simulink model "i_128w_2k_10_r306f"  (Simulink 7.0)
settings: Solver=ode45  StartTime=0.0  StopTime=100000  RelTol=1e-3
undefined symbols (not defined in the file or in its folder): iBOB, pfb_coeff_gen_calc
libraries: xbsIndex_r4 x946, casper_library x68, xps_library x29, xbsReplacements_r4 x12, simulink x1
(part 1 of 10)
settings Model: Creator=dsp  LastModifiedBy=dsp

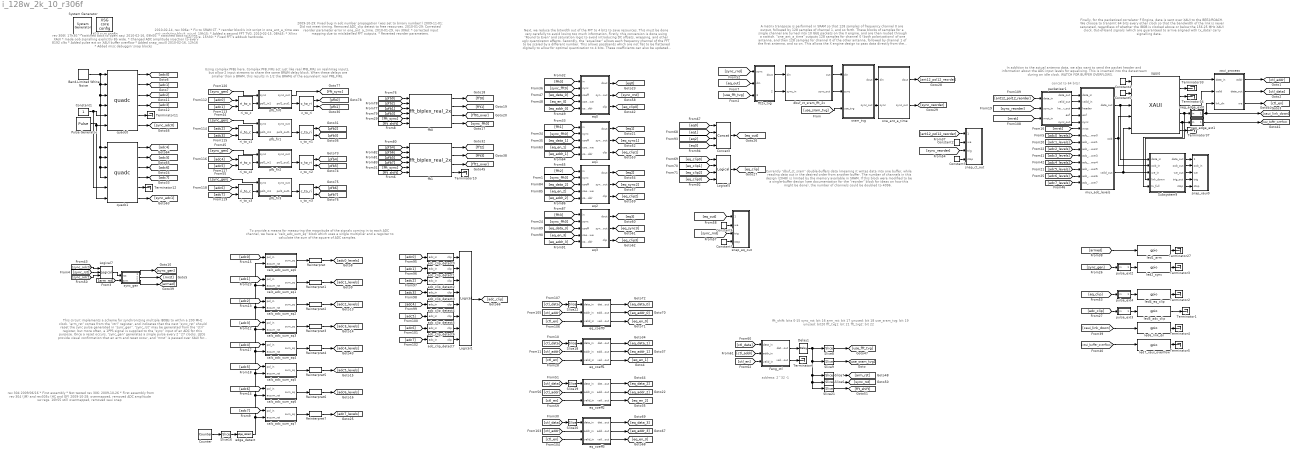
== system i_128w_2k_10_r306f ==
  note: 2010-02-14, rev 306e:
      |   * Fix to SRAM CT.
      |   * reorder block's init script in one_ant_a_time was not updating block. wierd.
      | 19h15:
      |   * Added a second FFT TVG.
      | 2010-02-15, 08h45:
      |   * Xilinx XAUI core.
      | 15h30:
      |   * Fixed FFT's addsub hardcode.
  note: This circuit implements a scheme for synchronizing
      | multiple IBOBs to within a 200 MHz clock.  "arm_rst"
      | comes from the "ctrl" register, and indicates that the
      | next "sync_rst" should reset the sync pulse generated
      | in "sync_gen".  "sync_rst" may be generated from
      | the "ctrl" register, but more often, a 1PPS signal is
      | supplied to the "sync" input of an ADC for this
      | purpose.  Once a reset occurs, "sync_gen" generates
      | a single pulse every 2^27 clocks.  LEDs provide visual
      | confirmation that an arm and reset occur, and "mrst"
      | is passed over XAUI for the purpose of informing
      | downstream logic in a packetized correlator that
      | a "master reset" has occurred.
  note: Using complex PFBs here.  Complex PFB_FIRs act just like real
      | PFB_FIRs on real/imag inputs, but  allow 2 input streams to
      | share the same BRAM delay block.  When these delays are smaller
      | than a BRAM, this results in 1/2 the BRAMs of the equivalent real
      | PFB_FIRs.
  note: To provide a means for measuring the magnitude of the signals
      | coming in to each ADC channel, we have a "calc_adc_sum_sq"
      | block which uses a single multiplier and a regsiter to calculate
      | the sum of the square of ADC samples.
  note: fft_shift: bits 0-15
      | sync_rst: bit 16
      | arm_rst: bit 17
      | unused: bit 18
      | use_sram_tvg: bit 19
      | unused: bit20
      | fft_tvg1: bit 21
      | fft_tvg2: bit 22
  note: address: 2^32 -1
  note: Finally, for the packetized correlator F Engine, data is sent over
      | XAUI to the BEE2/ROACH.  We choose to transmit 64 bits every other clock
      | so that the bandwidth of the link is never saturated, regardless of whether
      | the IBOB is clocked above or below the 156.25 MHz XAUI clock.
      | Out-of-band signals (which are guaranteed to arrive aligned with
      | tx_data) carry signalling data.
  note: In addition to the actual antenna data,
      | we also want to send the packet header
      | and information about the ADC input levels for equalising.
      | This is inserted into the datastream during an idle clock.
      | WATCH FOR BUFFER OVERFLOWS.
  note: concat to 64 bits!
  note: A matrix transpose is performed in SRAM so that 128 samples of frequency
      | channel 0 are output, followed by 128 samples of channel 1, and so forth.
      | These blocks of samples for a single channel are turned into 10 GbE packets
      | on the X engine, and are then routed through a swittch.  "one_ant_a_time"
      | outputs 128 samples for channel 0 (both polarizations) of one antenna,
      | and then 128 samples for channel 0 of the other antenna, followed by
      | channel 1 of the first antenna, and so on.  This allows the X engine design to
      | pass data directly from the XAUI into a packet containing 128 time samples
      | for 1 frequency from 1 antenna.
  note: Currently "dbuf_ct_sram" double-buffers data (meaning it writes data
      | into one buffer, while reading data out in the desired order from another
      | buffer.  The number of channels in this design (2048) is limited by the
      | memory available in SRAM.  If this block were modified to be a
      | single-buffer design (see documentation for the "reorder" block for
      | ideas on how this might be done), the number of channels could
      | be doubled to 4096.
  note: Next, we reduce the bitwidth out of the FFT to 4 bits to save resources.
      | This must be done very carefully to avoid losing too much information.
      | Firstly, this conversion is done using "Round to Even" and saturation
      | logic to avoid introducing DC offsets, wrapping, and other ugly quantizaton
      | effects.  Secondly, the "equalizer" allows each frequency channel of the
      | FFT to be scaled by a different number.  This allows passbands which are
      | not flat to be flattened digitally to allow for optimal quantization to 4 bits.
      | These coefficients can also be updated dynamically for gain control.
      | Coefficients can be dynamically written into the "equalizer" by
      | specifying the channel ("coeff_addr") and the value of the
      | coefficient ("coeff"), and then using "coeff_en" to write the
      | new coefficient into the equalization table.
  note: rev 304 2009/06/16
      | * First assembly
      | * Not tested
      |
      | rev 306: 2009-10-26
      | * First assembly from rev 304 (JM) and rev305c (HC and GF)
      |
      | 2009-10-28: overmapped, removed ADC amplitude sw regs.
      | 10h55 still overmapped, removed xaui snap
  note: 2009-10-29: Fixed bug in adc number propagation (was set to binary number!)
      | 2009-11-01: Did not meet timing. Removed ADC_clip detect to free resources.
      | 2010-01-29: Corrected reorder parameter error in one_ant_a_time.
      |
      | 2010-01-29, rev 306d:
      |   * corrected input mapping due to mislabelled FFT outputs.
      |   * Reverted reorder parameters.
  note: rev 306f, 17h30:
      |   * switched back to open xaui
      | 2010-02-16, 09h00:
      |   * switched back to Xilinx XAUI
      |   * made oob signalling explicitly 8b wide.
      |   * Changed ADC amplitude injection to every 8192 clks
      |   * Added pulse ext on XAUI buffer overflow
      |   * Added snap_xaui0
      | 2010-02-16, 12h16
      |   * Added misc debuggin' snap blocks
  " System Generator" : xbsIndex_r4/ System Generator  Tag=genX  SystemSampleTime=-1  xilinxfamily=virtex2p  part=xc2vp50  speed=-7  package=ff1152  synthesis_tool=XST  clock_wrapper=Clock Enables  directory=./i_128w_2k_10_r306f/sysgen  testbench=off  simulink_period=1  sysclk_period=5  dcm_input_clock_period=100  incr_netlist=off  trim_vbits=Everywhere in SubSystem  dbl_ovrd=According to Block Masks  core_generation=According to Block Masks  run_coregen=off  deprecated_control=off  eval_field=0  block_type=sysgen
      settings: block_version=10.1.3
  Band-Limited White Noise : simulink/Sources/Band-Limited White Noise  SystemSampleTime=-1  Cov=[0.1]  Ts=0.1  seed=[23341]
  Concat3 : xbsIndex_r4/Concat  num_inputs=4  dbl_ovrd=off  block_type=concat
      settings: block_version=10.1.3
  Constant1 : Constant  OutDataType=sfix(16)  OutScaling=2^0
  Constant2 : xbsIndex_r4/Constant  arith_type=Boolean  const=1  n_bits=1  bin_pt=0  explicit_period=on  period=1  equ=P=C  opselect=C  inp2=PCIN>>17  opr=+  inp1=P  carry=CIN  dbl_ovrd=off  block_type=constant
  Constant3 : xbsIndex_r4/Constant  arith_type=Boolean  const=0  n_bits=1  bin_pt=0  explicit_period=on  period=1  equ=P=C  opselect=C  inp2=PCIN>>17  opr=+  inp1=P  carry=CIN  dbl_ovrd=off  block_type=constant
  Constant4 : xbsIndex_r4/Constant  arith_type=Unsigned  const=1  n_bits=1  bin_pt=0  explicit_period=on  period=1  equ=P=C  opselect=C  inp2=PCIN>>17  opr=+  inp1=P  carry=CIN  dbl_ovrd=off  block_type=constant
  Constant5 : xbsIndex_r4/Constant  arith_type=Unsigned  const=0  n_bits=1  bin_pt=0  explicit_period=on  period=1  equ=P=C  opselect=C  inp2=PCIN>>17  opr=+  inp1=P  carry=CIN  dbl_ovrd=off  block_type=constant
  Constant6 : xbsIndex_r4/Constant  arith_type=Boolean  const=1  n_bits=1  bin_pt=0  explicit_period=on  period=1  equ=P=C  opselect=C  inp2=PCIN>>17  opr=+  inp1=P  carry=CIN  dbl_ovrd=off  block_type=constant
  Constant7 : xbsIndex_r4/Constant  arith_type=Boolean  const=0  n_bits=1  bin_pt=0  explicit_period=on  period=1  equ=P=C  opselect=C  inp2=PCIN>>17  opr=+  inp1=P  carry=CIN  dbl_ovrd=off  block_type=constant
  Counter : xbsIndex_r4/Counter  cnt_type=Free Running  cnt_to=Inf  operation=Up  start_count=0  cnt_by_val=1  arith_type=Unsigned  n_bits=16  bin_pt=0  load_pin=off  rst=off  en=off  explicit_period=off  period=1  dbl_ovrd=off  use_behavioral_HDL=off  use_rpm=on  implementation=Fabric  block_type=counter
      settings: xl_area=[0, 0, 0, 0, 0, 0, 0]
  Delay1 : xbsIndex_r4/Delay  en=off  latency=1  dbl_ovrd=off  reg_retiming=off  block_type=delay
      settings: xl_area=[0, 0, 0, 0, 0, 0, 0]
  Feng_ctl : Subsystem  mask{addr_offset=8192}
      mask prompts: addr_offset "Address"
      mask init:
      | start_addr = (addr_offset);
      | fmtstr = sprintf('Mapped address: %d', start_addr);
      | set_param(gcb, 'AttributesFormatString', fmtstr);
      settings: AttributesFormatString=Mapped address: 8192
  Logical1 : xbsIndex_r4/Logical  logical_function=OR  inputs=8  en=off  latency=1  precision=Full  arith_type=Unsigned  n_bits=8  bin_pt=2  align_bp=on  dbl_ovrd=off  block_type=logical
      settings: xl_area=[0, 0, 0, 0, 0, 0, 0]
  Logical5 : xbsIndex_r4/Logical  logical_function=OR  inputs=4  en=off  latency=0  precision=Full  arith_type=Unsigned  n_bits=8  bin_pt=2  align_bp=on  dbl_ovrd=off  block_type=logical
      settings: xl_area=[0, 0, 0, 0, 0, 0, 0]
  Logical7 : xbsIndex_r4/Logical  logical_function=OR  inputs=3  en=off  latency=1  precision=Full  arith_type=Unsigned  n_bits=8  bin_pt=2  align_bp=on  dbl_ovrd=off  block_type=logical
      settings: xl_area=[0, 0, 0, 0, 0, 0, 0]
  Pulse Generator : DiscretePulseGenerator  Period=2^27
  Reinterpret{,1..7} (8 alike) : xbsIndex_r4/Reinterpret  force_arith_type=on  arith_type=Unsigned  force_bin_pt=on  bin_pt=0  block_type=reinterpret
      settings: infoedit="Changes signal type without altering the binary representation.   You can changed the signal between signed and unsigned, and relocate the binary point.<P><P>Hardware notes: In hardware this block costs nothing.<P><P>Example:  Suppose the input is 6 bits wide, signed, with 2 fractional bits, and the output is forced to unsigned with 0 fractional bits.  Then an input of -2.0 (1110.00 in binary 2's complement) becomes an output of 56 (111000 in binary)."  block_version=10.1.3
  Slice16 : xbsIndex_r4/Slice  nbits=1  boolean_output=on  mode=Upper Bit Location + Width  bit1=0  base1=MSB of Input  bit0=19  base0=LSB of Input  dbl_ovrd=off  block_type=slice
      settings: infoedit="Extracts a given range of bits from each input sample and presents it at the output.  The output type is ordinarily unsigned with binary point at zero, but can be Boolean when the slice is one bit wide.<P><P>Hardware notes: In hardware this block costs nothing."  block_version=10.1.3
  Slice{18..20,22} (4 alike) : xbsIndex_r4/Slice  nbits=17  boolean_output=off  mode=Lower Bit Location + Width  bit1=0  base1=MSB of Input  bit0=0  base0=LSB of Input  dbl_ovrd=off  block_type=slice
      settings: infoedit="Extracts a given range of bits from each input sample and presents it at the output.  The output type is ordinarily unsigned with binary point at zero, but can be Boolean when the slice is one bit wide.<P><P>Hardware notes: In hardware this block costs nothing."  block_version=10.1.3
  Slice21 : xbsIndex_r4/Slice  nbits=16  boolean_output=off  mode=Lower Bit Location + Width  bit1=0  base1=MSB of Input  bit0=0  base0=LSB of Input  dbl_ovrd=off  block_type=slice
      settings: infoedit="Extracts a given range of bits from each input sample and presents it at the output.  The output type is ordinarily unsigned with binary point at zero, but can be Boolean when the slice is one bit wide.<P><P>Hardware notes: In hardware this block costs nothing."  block_version=10.1.3
  Slice6 : xbsIndex_r4/Slice  nbits=1  boolean_output=on  mode=Lower Bit Location + Width  bit1=0  base1=MSB of Input  bit0=16  base0=LSB of Input  dbl_ovrd=off  block_type=slice
      settings: infoedit="Extracts a given range of bits from each input sample and presents it at the output.  The output type is ordinarily unsigned with binary point at zero, but can be Boolean when the slice is one bit wide.<P><P>Hardware notes: In hardware this block costs nothing."  block_version=10.1.3
  Slice7 : xbsIndex_r4/Slice  nbits=1  boolean_output=on  mode=Lower Bit Location + Width  bit1=0  base1=MSB of Input  bit0=17  base0=LSB of Input  dbl_ovrd=off  block_type=slice
      settings: infoedit="Extracts a given range of bits from each input sample and presents it at the output.  The output type is ordinarily unsigned with binary point at zero, but can be Boolean when the slice is one bit wide.<P><P>Hardware notes: In hardware this block costs nothing."  block_version=10.1.3
  Slice8 : xbsIndex_r4/Slice  nbits=2  boolean_output=off  mode=Lower Bit Location + Width  bit1=0  base1=MSB of Input  bit0=21  base0=LSB of Input  dbl_ovrd=off  block_type=slice
      settings: infoedit="Extracts a given range of bits from each input sample and presents it at the output.  The output type is ordinarily unsigned with binary point at zero, but can be Boolean when the slice is one bit wide.<P><P>Hardware notes: In hardware this block costs nothing."  block_version=10.1.3
  Slice9 : xbsIndex_r4/Slice  nbits=1  boolean_output=off  mode=Lower Bit Location + Width  bit1=0  base1=MSB of Input  bit0=19  base0=LSB of Input  dbl_ovrd=off  block_type=slice
      settings: infoedit="Extracts a given range of bits from each input sample and presents it at the output.  The output type is ordinarily unsigned with binary point at zero, but can be Boolean when the slice is one bit wide.<P><P>Hardware notes: In hardware this block costs nothing."  block_version=10.1.3
  Subsystem9 : Subsystem
  Terminator{1..6,10..12,27,33..34,37} (13 alike) : Terminator
  XAUI0 : xps_library/XAUI  Tag=xps:xaui  SystemSampleTime=-1  demux=1  port=iBOB:0  open_phy=off  show_param=off  pre_emph=3  swing=800
      link override convert_tx_data: n_bits=64
      link override convert_tx_outofband: n_bits=8
      link override i_128w_2k_10_r304_XAUI0_rx_data: n_bits=64
      link override i_128w_2k_10_r304_XAUI0_rx_outofband: n_bits=8
      link override i_128w_2k_10_r306_XAUI0_rx_data: n_bits=64
      link override i_128w_2k_10_r306_XAUI0_rx_outofband: n_bits=8
      link override i_128w_2k_10_r306e_XAUI0_rx_data: n_bits=64
      link override i_128w_2k_10_r306e_XAUI0_rx_outofband: n_bits=8
      link override i_128w_2k_10_r306f_XAUI0_rx_data: n_bits=64
      link override i_128w_2k_10_r306f_XAUI0_rx_outofband: n_bits=8
      link override i_128w_4k_10_150_r305a_XAUI0_rx_data: n_bits=64
      link override i_128w_4k_10_150_r305a_XAUI0_rx_outofband: n_bits=8
      link override i_128w_4k_10_150_r305b_XAUI0_rx_data: n_bits=64
      link override i_128w_4k_10_150_r305b_XAUI0_rx_outofband: n_bits=8
      link override i_128w_4k_10_200_r304_XAUI0_rx_data: n_bits=64
      link override i_128w_4k_10_200_r304_XAUI0_rx_outofband: n_bits=8
      link override i_128w_4k_10_200_r305a_XAUI0_rx_data: n_bits=64
      link override i_128w_4k_10_200_r305a_XAUI0_rx_outofband: n_bits=8
      link override temp_feng_XAUI0_rx_data: n_bits=64
      link override temp_feng_XAUI0_rx_outofband: n_bits=8
  XSG core config : xps_library/XSG core config  Tag=xps:xsg  SystemSampleTime=-1  hw_sys=iBOB  ibob_linux=off  clk_src=adc0_clk  iBOB_clk_src=adc0_clk  BEE2_ctrl_clk_src=sys_clk  BEE2_usr_clk_src=sys_clk  ROACH_clk_src=arb_clk  CORR_clk_src=sys_clk  gpio_clk_io_group=iBOB:sma  gpio_clk_bit_index=0  clk_rate=200  sample_period=1  synthesis_tool=XST  mpc_type=powerpc405
  adc_clip_detect0 : Subsystem  mask{n_bits=8}
      mask prompts: n_bits "Number of ADC bits"
  adc_clip_detect1 : Subsystem  mask{n_bits=8}
      mask prompts: n_bits "Number of ADC bits"
  adc_clip_detect2 : Subsystem  mask{n_bits=8}
      mask prompts: n_bits "Number of ADC bits"
  adc_clip_detect3 : Subsystem  mask{n_bits=8}
      mask prompts: n_bits "Number of ADC bits"
  adc_clip_detect4 : Subsystem  mask{n_bits=8}
      mask prompts: n_bits "Number of ADC bits"
  adc_clip_detect5 : Subsystem  mask{n_bits=8}
      mask prompts: n_bits "Number of ADC bits"
  adc_clip_detect6 : Subsystem  mask{n_bits=8}
      mask prompts: n_bits "Number of ADC bits"
  adc_clip_detect7 : Subsystem  mask{n_bits=8}
      mask prompts: n_bits "Number of ADC bits"
  c_to_ri{,1..3} (4 alike) : casper_library/Misc/c_to_ri  SystemSampleTime=-1  n_bits=18  bin_pt=17
      settings: AttributesFormatString=18_17 r/i
  calc_adc_sum_sq0 : Subsystem
  calc_adc_sum_sq1 : Subsystem
  calc_adc_sum_sq2 : Subsystem
  calc_adc_sum_sq3 : Subsystem
  calc_adc_sum_sq4 : Subsystem
  calc_adc_sum_sq5 : Subsystem
  calc_adc_sum_sq6 : Subsystem
  calc_adc_sum_sq7 : Subsystem
  dbuf_ct_sram_fft_2x : Subsystem  mask{length=11, numSpecs=7}
      mask prompts: length "Length of Spectrums (2^?) (FFT_real_2x vector length)"; numSpecs "Number of Spectrums (2^?) (pkt size in 16bit complex dual-pol words)"
      mask help: Sram transpose using double buffering method, maximum size is 256 spectrums by 2048 channels!!
  edge_detect : casper_library/Misc/edge_detect  SystemSampleTime=-1  edge=Rising  polarity=Active High  x_in=[0 0.08 0.08 0.16 0.16 0.24 0.24 0.32 0.32 0.4]  y_in="[-1 -1  1  1  1  1  1  1  1  1]"  x_out=[0.6 0.68 0.68 0.76 0.76 0.84 0.84 0.92 0.92 1]  y_out="[-1 -1  1  1 -1 -1 -1 -1 -1 -1]"
      settings: AttributesFormatString=|
      | rising edges
      | active high
  eq0 : Subsystem
  eq1 : Subsystem
  eq2 : Subsystem
  eq3 : Subsystem
  eq_coeff0 : Subsystem  mask{addr_width=6, addr_offset=0}
      mask prompts: addr_width "Number of addresses (2^?)"; addr_offset "Address block offset (multiple of above)"
      mask init:
      | start_addr = 2^addr_width*(addr_offset);
      | end_addr = start_addr + 2^addr_width - 1;
      | fmtstr = sprintf('Mapped address range: %d-%d', start_addr,end_addr);
      | set_param(gcb, 'AttributesFormatString', fmtstr);
      settings: AttributesFormatString=Mapped address range: 0-63
  eq_coeff1 : Subsystem  mask{addr_width=6, addr_offset=1}
      mask prompts: addr_width "Number of addresses (2^?)"; addr_offset "Address block offset (multiple of above)"
      mask init: same as i_128w_2k_10_r306f/eq_coeff0
      settings: AttributesFormatString=Mapped address range: 64-127
  eq_coeff2 : Subsystem  mask{addr_width=6, addr_offset=2}
      mask prompts: addr_width "Number of addresses (2^?)"; addr_offset "Address block offset (multiple of above)"
      mask init: same as i_128w_2k_10_r306f/eq_coeff0
      settings: AttributesFormatString=Mapped address range: 128-191
  eq_coeff3 : Subsystem  mask{addr_width=6, addr_offset=3}
      mask prompts: addr_width "Number of addresses (2^?)"; addr_offset "Address block offset (multiple of above)"
      mask init: same as i_128w_2k_10_r306f/eq_coeff0
      settings: AttributesFormatString=Mapped address range: 192-255
  fft0 : casper_library/FFTs/fft_biplex_real_2x  SystemSampleTime=-1  FFTSize=11  input_bit_width=18  coeff_bit_width=18  quantization="Round  (unbiased: Even Values)"  overflow=Wrap  add_latency=1  mult_latency=3  bram_latency=2  arch=Virtex2Pro  opt_target=Multipliers  coeffs_bit_limit=7  delays_bit_limit=8  specify_mult=on  mult_spec=[1 1 1 1 1 1 1 1 1 1 1]  dsp48_adders=off
      settings: AttributesFormatString=FFTSize=11
  fft1 : casper_library/FFTs/fft_biplex_real_2x  SystemSampleTime=-1  FFTSize=11  input_bit_width=18  coeff_bit_width=18  quantization="Round  (unbiased: Even Values)"  overflow=Wrap  add_latency=1  mult_latency=3  bram_latency=2  arch=Virtex2Pro  opt_target=Multipliers  coeffs_bit_limit=7  delays_bit_limit=8  specify_mult=on  mult_spec=[1 1 1 1 1 1 1 1 1 1 1]  dsp48_adders=off
      settings: AttributesFormatString=FFTSize=11
  fft2x_tvg : Subsystem  mask{length=11}
      mask prompts: length "FFT_real_2x vector length (2^?)"
  led1_arm : xps_library/gpio  Tag=xps:gpio  SystemSampleTime=-1  io_group=iBOB:led  io_dir=out  arith_type=Boolean  bitwidth=1  bin_pt=0  bit_index=1  sample_period=1  use_single_ended=off  use_ddr=off  reg_iob=on  reg_clk_phase=0  termination=None
      link override convert: arith_type=Boolean  n_bits=1  bin_pt=0
  led2_sync : xps_library/gpio  Tag=xps:gpio  SystemSampleTime=-1  io_group=iBOB:led  io_dir=out  arith_type=Boolean  bitwidth=1  bin_pt=0  bit_index=2  sample_period=1  use_single_ended=off  use_ddr=off  reg_iob=on  reg_clk_phase=0  termination=None
      link override convert: arith_type=Boolean  n_bits=1  bin_pt=0
  led4_eq_clip : xps_library/gpio  Tag=xps:gpio  SystemSampleTime=-1  io_group=iBOB:led  io_dir=out  arith_type=Boolean  bitwidth=1  bin_pt=0  bit_index=4  sample_period=1  use_single_ended=off  use_ddr=off  reg_iob=on  reg_clk_phase=0  termination=None
      link override convert: arith_type=Boolean  n_bits=1  bin_pt=0
  led5_adc_clip : xps_library/gpio  Tag=xps:gpio  SystemSampleTime=-1  io_group=iBOB:led  io_dir=out  arith_type=Boolean  bitwidth=1  bin_pt=0  bit_index=5  sample_period=1  use_single_ended=off  use_ddr=off  reg_iob=on  reg_clk_phase=0  termination=None
      link override convert: arith_type=Boolean  n_bits=1  bin_pt=0
  led6_link_dn : xps_library/gpio  Tag=xps:gpio  SystemSampleTime=-1  io_group=iBOB:led  io_dir=out  arith_type=Unsigned  bitwidth=1  bin_pt=0  bit_index=6  sample_period=1  use_single_ended=off  use_ddr=off  reg_iob=on  reg_clk_phase=0  termination=None
      link override convert: arith_type=Unsigned  n_bits=1  bin_pt=0
  led7_xaui_overlfow : xps_library/gpio  Tag=xps:gpio  SystemSampleTime=-1  io_group=iBOB:led  io_dir=out  arith_type=Unsigned  bitwidth=1  bin_pt=0  bit_index=7  sample_period=1  use_single_ended=off  use_ddr=off  reg_iob=on  reg_clk_phase=0  termination=None
      link override convert: arith_type=Unsigned  n_bits=1  bin_pt=0
  mux_adc_levels : Subsystem
  neg_edge_ext0 : Subsystem  mask{pulse_len=2^27}
      mask prompts: pulse_len "Length of Pulse"
      mask init:
      | bits = ceil(log2(pulse_len+1));
  neg_edge_ext1 : Subsystem  mask{pulse_len=2^23}
      mask prompts: pulse_len "Length of Pulse"
      mask init:
      | bits = ceil(log2(pulse_len+1));
  one_ant_a_time : Subsystem
  packetiser1 : Subsystem  mask{nwrd_bits=5, ant_bits=2}
      mask prompts: nwrd_bits "Payload length: (in 64bit words) (2^n)"; ant_bits "Number of antennas on this link (2^n)"
      mask help: Package 32 bit data into 64 bits and identify data as coming from antenna 0 or 1
  pfb_fir0 : Subsystem  AncestorBlock=casper_library/PFBs/pfb_fir  mask(pfb_fir){PFBSize=11, TotalTaps=4, WindowType=hamming, n_inputs=0, MakeBiplex=0, BitWidthIn=8, BitWidthOut=18, CoeffBitWidth=8, CoeffDistMem=0, add_latency=1, mult_latency=2, bram_latency=3, quantization=Round  (unbiased: Even Values), fwidth=1, specify_mult=off, mult_spec=[0 1 2 0]}
      mask prompts: PFBSize "Size of PFB: (2^? pnts)"; TotalTaps "Total Number of Taps:"; WindowType "Windowing Function:"; n_inputs "Number of Simultaneous Inputs: (2^?)"; MakeBiplex "Make Biplex"; BitWidthIn "Input Bitwidth:"; BitWidthOut "Output Bitwidth:"; CoeffBitWidth "Coefficient Bitwidth:"; CoeffDistMem "Use Distributed Memory for Coeffs"; add_latency "Add Latency"; mult_latency "Mult Latency"; bram_latency "BRAM Latency"; quantization "Quantization Behavior"; fwidth "Bin Width Scaling (normal=1)"; specify_mult "Specify multiplier use (embedded if not specified)"; mult_spec "Multiplier specification (0=core, 1=embedded, 2=behavioural) (left=1st tap)"
      mask init:
      | pfb_fir_init(gcb, ...
      |     'PFBSize', PFBSize, ...
      |     'TotalTaps', TotalTaps, ...
      |     'WindowType', WindowType, ...
      |     'n_inputs', n_inputs, ...
      |     'MakeBiplex', MakeBiplex, ...
      |     'BitWidthIn', BitWidthIn, ...
      |     'BitWidthOut', BitWidthOut, ...
      |     'CoeffBitWidth', CoeffBitWidth, ...
      |     'CoeffDistMem', CoeffDistMem, ...
      |     'add_latency', add_latency, ...
      |     'mult_latency', mult_latency, ...
      |     'bram_latency', bram_latency, ...
      |     'quantization', quantization, ...
      |     'fwidth', fwidth,...
      |     'specify_mult', specify_mult,...
      |     'mult_spec', mult_spec);
      settings: AttributesFormatString=taps=4, add_latency=1
      mask Help: eval('xlWeb([getenv(''MLIB_ROOT''), ''\doc\htmlblocks\sp_pfb_fir\sp_pfb_fir.html''])')
      mask StyleString: edit,edit,popup(bartlett|barthannwin|blackman|blackmanharris|bohamwin|chebwin|flattopwin|gausswin|hamming|hann|kaiser|nuttallwin|parzenwin|rectwin|tukeywin|triang|userwindow),edit,edit,edit,edit,edit,edit,edit,edit,edit,popup(Truncate|Round  (unbiased: +/- Inf)|Round  (unbiased: Even Values)),edit,checkbox,edit
      mask CallbackString:
      | |num_taps = eval(get_param(gcb, 'TotalTaps'));
      | old_vec = eval(get_param(gcb, 'mult_spec'));
      | 
      | vec = ones(1,num_taps);
      | old_size = length(old_vec);
      | 
      | if(old_size <= num_taps),
      |     size = old_size;
      | else,
      |     size = num_taps;
      | end
      | 
      | for n = 1:size, vec(n) = old_vec(n); end
      | set_param(gcb, 'mult_spec', mat2str(vec));|||||||||||||specify_mult = get_param(gcb,'specify_mult');
      | if( strcmp(specify_mult,'off')),
      |     set_param(gcb, 'MaskEnables', {'on','on','on','on','on','on','on','on','on','on','on','on','on','on','on','off'});
      | else
      |     set_param(gcb, 'MaskEnables', {'on','on','on','on','on','on','on','on','on','on','on','on','on','on','on','on'});
      | end
      | 
      | |vec = eval( get_param(gcb, 'mult_spec'));
      | vec_size = length(vec);
      | num_taps = eval( get_param(gcb, 'TotalTaps'));
      | new_vec = ones(1, num_taps);
      | 
      | if(vec_size <= num_taps), size = vec_size;
      | else size = num_taps;
      | end
      | 
      | for n=1:size
      |     new_vec(n) = vec(n);
      | end
      | set_param(gcb, 'mult_spec', mat2str(new_vec));
  pfb_fir1 : Subsystem  AncestorBlock=casper_library/PFBs/pfb_fir  mask(pfb_fir){PFBSize=11, TotalTaps=4, WindowType=hamming, n_inputs=0, MakeBiplex=0, BitWidthIn=8, BitWidthOut=18, CoeffBitWidth=8, CoeffDistMem=0, add_latency=1, mult_latency=2, bram_latency=3, quantization=Round  (unbiased: Even Values), fwidth=1, specify_mult=off, mult_spec=[0 1 2 0]}
      mask prompts: PFBSize "Size of PFB: (2^? pnts)"; TotalTaps "Total Number of Taps:"; WindowType "Windowing Function:"; n_inputs "Number of Simultaneous Inputs: (2^?)"; MakeBiplex "Make Biplex"; BitWidthIn "Input Bitwidth:"; BitWidthOut "Output Bitwidth:"; CoeffBitWidth "Coefficient Bitwidth:"; CoeffDistMem "Use Distributed Memory for Coeffs"; add_latency "Add Latency"; mult_latency "Mult Latency"; bram_latency "BRAM Latency"; quantization "Quantization Behavior"; fwidth "Bin Width Scaling (normal=1)"; specify_mult "Specify multiplier use (embedded if not specified)"; mult_spec "Multiplier specification (0=core, 1=embedded, 2=behavioural) (left=1st tap)"
      mask init: same as i_128w_2k_10_r306f/pfb_fir0
      settings: AttributesFormatString=taps=4, add_latency=1
      mask Help: eval('xlWeb([getenv(''MLIB_ROOT''), ''\doc\htmlblocks\sp_pfb_fir\sp_pfb_fir.html''])')
      mask StyleString: edit,edit,popup(bartlett|barthannwin|blackman|blackmanharris|bohamwin|chebwin|flattopwin|gausswin|hamming|hann|kaiser|nuttallwin|parzenwin|rectwin|tukeywin|triang|userwindow),edit,edit,edit,edit,edit,edit,edit,edit,edit,popup(Truncate|Round  (unbiased: +/- Inf)|Round  (unbiased: Even Values)),edit,checkbox,edit
      mask CallbackString:
      | |num_taps = eval(get_param(gcb, 'TotalTaps'));
      | old_vec = eval(get_param(gcb, 'mult_spec'));
      | 
      | vec = ones(1,num_taps);
      | old_size = length(old_vec);
      | 
      | if(old_size <= num_taps),
      |     size = old_size;
      | else,
      |     size = num_taps;
      | end
      | 
      | for n = 1:size, vec(n) = old_vec(n); end
      | set_param(gcb, 'mult_spec', mat2str(vec));|||||||||||||specify_mult = get_param(gcb,'specify_mult');
      | if( strcmp(specify_mult,'off')),
      |     set_param(gcb, 'MaskEnables', {'on','on','on','on','on','on','on','on','on','on','on','on','on','on','on','off'});
      | else
      |     set_param(gcb, 'MaskEnables', {'on','on','on','on','on','on','on','on','on','on','on','on','on','on','on','on'});
      | end
      | 
      | |vec = eval( get_param(gcb, 'mult_spec'));
      | vec_size = length(vec);
      | num_taps = eval( get_param(gcb, 'TotalTaps'));
      | new_vec = ones(1, num_taps);
      | 
      | if(vec_size <= num_taps), size = vec_size;
      | else size = num_taps;
      | end
      | 
      | for n=1:size
      |     new_vec(n) = vec(n);
      | end
      | set_param(gcb, 'mult_spec', mat2str(new_vec));
  pfb_fir2 : Subsystem  AncestorBlock=casper_library/PFBs/pfb_fir  mask(pfb_fir){PFBSize=11, TotalTaps=4, WindowType=hamming, n_inputs=0, MakeBiplex=0, BitWidthIn=8, BitWidthOut=18, CoeffBitWidth=8, CoeffDistMem=0, add_latency=1, mult_latency=2, bram_latency=3, quantization=Round  (unbiased: Even Values), fwidth=1, specify_mult=off, mult_spec=[0 1 2 0]}
      mask prompts: PFBSize "Size of PFB: (2^? pnts)"; TotalTaps "Total Number of Taps:"; WindowType "Windowing Function:"; n_inputs "Number of Simultaneous Inputs: (2^?)"; MakeBiplex "Make Biplex"; BitWidthIn "Input Bitwidth:"; BitWidthOut "Output Bitwidth:"; CoeffBitWidth "Coefficient Bitwidth:"; CoeffDistMem "Use Distributed Memory for Coeffs"; add_latency "Add Latency"; mult_latency "Mult Latency"; bram_latency "BRAM Latency"; quantization "Quantization Behavior"; fwidth "Bin Width Scaling (normal=1)"; specify_mult "Specify multiplier use (embedded if not specified)"; mult_spec "Multiplier specification (0=core, 1=embedded, 2=behavioural) (left=1st tap)"
      mask init: same as i_128w_2k_10_r306f/pfb_fir0
      settings: AttributesFormatString=taps=4, add_latency=1
      mask Help: eval('xlWeb([getenv(''MLIB_ROOT''), ''\doc\htmlblocks\sp_pfb_fir\sp_pfb_fir.html''])')
      mask StyleString: edit,edit,popup(bartlett|barthannwin|blackman|blackmanharris|bohamwin|chebwin|flattopwin|gausswin|hamming|hann|kaiser|nuttallwin|parzenwin|rectwin|tukeywin|triang|userwindow),edit,edit,edit,edit,edit,edit,edit,edit,edit,popup(Truncate|Round  (unbiased: +/- Inf)|Round  (unbiased: Even Values)),edit,checkbox,edit
      mask CallbackString:
      | |num_taps = eval(get_param(gcb, 'TotalTaps'));
      | old_vec = eval(get_param(gcb, 'mult_spec'));
      | 
      | vec = ones(1,num_taps);
      | old_size = length(old_vec);
      | 
      | if(old_size <= num_taps),
      |     size = old_size;
      | else,
      |     size = num_taps;
      | end
      | 
      | for n = 1:size, vec(n) = old_vec(n); end
      | set_param(gcb, 'mult_spec', mat2str(vec));|||||||||||||specify_mult = get_param(gcb,'specify_mult');
      | if( strcmp(specify_mult,'off')),
      |     set_param(gcb, 'MaskEnables', {'on','on','on','on','on','on','on','on','on','on','on','on','on','on','on','off'});
      | else
      |     set_param(gcb, 'MaskEnables', {'on','on','on','on','on','on','on','on','on','on','on','on','on','on','on','on'});
      | end
      | 
      | |vec = eval( get_param(gcb, 'mult_spec'));
      | vec_size = length(vec);
      | num_taps = eval( get_param(gcb, 'TotalTaps'));
      | new_vec = ones(1, num_taps);
      | 
      | if(vec_size <= num_taps), size = vec_size;
      | else size = num_taps;
      | end
      | 
      | for n=1:size
      |     new_vec(n) = vec(n);
      | end
      | set_param(gcb, 'mult_spec', mat2str(new_vec));
  pfb_fir3 : Subsystem  AncestorBlock=casper_library/PFBs/pfb_fir  mask(pfb_fir){PFBSize=11, TotalTaps=4, WindowType=hamming, n_inputs=0, MakeBiplex=0, BitWidthIn=8, BitWidthOut=18, CoeffBitWidth=8, CoeffDistMem=0, add_latency=1, mult_latency=2, bram_latency=3, quantization=Round  (unbiased: Even Values), fwidth=1, specify_mult=off, mult_spec=[0 1 2 0]}
      mask prompts: PFBSize "Size of PFB: (2^? pnts)"; TotalTaps "Total Number of Taps:"; WindowType "Windowing Function:"; n_inputs "Number of Simultaneous Inputs: (2^?)"; MakeBiplex "Make Biplex"; BitWidthIn "Input Bitwidth:"; BitWidthOut "Output Bitwidth:"; CoeffBitWidth "Coefficient Bitwidth:"; CoeffDistMem "Use Distributed Memory for Coeffs"; add_latency "Add Latency"; mult_latency "Mult Latency"; bram_latency "BRAM Latency"; quantization "Quantization Behavior"; fwidth "Bin Width Scaling (normal=1)"; specify_mult "Specify multiplier use (embedded if not specified)"; mult_spec "Multiplier specification (0=core, 1=embedded, 2=behavioural) (left=1st tap)"
      mask init: same as i_128w_2k_10_r306f/pfb_fir0
      settings: AttributesFormatString=taps=4, add_latency=1
      mask Help: eval('xlWeb([getenv(''MLIB_ROOT''), ''\doc\htmlblocks\sp_pfb_fir\sp_pfb_fir.html''])')
      mask StyleString: edit,edit,popup(bartlett|barthannwin|blackman|blackmanharris|bohamwin|chebwin|flattopwin|gausswin|hamming|hann|kaiser|nuttallwin|parzenwin|rectwin|tukeywin|triang|userwindow),edit,edit,edit,edit,edit,edit,edit,edit,edit,popup(Truncate|Round  (unbiased: +/- Inf)|Round  (unbiased: Even Values)),edit,checkbox,edit
      mask CallbackString:
      | |num_taps = eval(get_param(gcb, 'TotalTaps'));
      | old_vec = eval(get_param(gcb, 'mult_spec'));
      | 
      | vec = ones(1,num_taps);
      | old_size = length(old_vec);
      | 
      | if(old_size <= num_taps),
      |     size = old_size;
      | else,
      |     size = num_taps;
      | end
      | 
      | for n = 1:size, vec(n) = old_vec(n); end
      | set_param(gcb, 'mult_spec', mat2str(vec));|||||||||||||specify_mult = get_param(gcb,'specify_mult');
      | if( strcmp(specify_mult,'off')),
      |     set_param(gcb, 'MaskEnables', {'on','on','on','on','on','on','on','on','on','on','on','on','on','on','on','off'});
      | else
      |     set_param(gcb, 'MaskEnables', {'on','on','on','on','on','on','on','on','on','on','on','on','on','on','on','on'});
      | end
      | 
      | |vec = eval( get_param(gcb, 'mult_spec'));
      | vec_size = length(vec);
      | num_taps = eval( get_param(gcb, 'TotalTaps'));
      | new_vec = ones(1, num_taps);
      | 
      | if(vec_size <= num_taps), size = vec_size;
      | else size = num_taps;
      | end
      | 
      | for n=1:size
      |     new_vec(n) = vec(n);
      | end
      | set_param(gcb, 'mult_spec', mat2str(new_vec));
  pulse_ext2 : Subsystem  mask{pulse_len=2^23}
      mask prompts: pulse_len "Length of Pulse"
      mask init:
      | bits = ceil(log2(pulse_len+1));
  pulse_ext3 : Subsystem  mask{pulse_len=2^23}
      mask prompts: pulse_len "Length of Pulse"
      mask init:
      | bits = ceil(log2(pulse_len+1));
  pulse_ext4 : Subsystem  mask{pulse_len=2^23}
      mask prompts: pulse_len "Length of Pulse"
      mask init:
      | bits = ceil(log2(pulse_len+1));
  quadc0 : xps_library/quadc  Tag=xps:quadc  SystemSampleTime=-1  adc_brd=0  adc_clk_rate=200
  quadc1 : xps_library/quadc  Tag=xps:quadc  SystemSampleTime=-1  adc_brd=1  adc_clk_rate=200
  ri_to_c{,1..3} (4 alike) : casper_library/Misc/ri_to_c  SystemSampleTime=-1
  snap_ct_out : Subsystem  mask{nsamples=13}
      mask prompts: nsamples "Number of Samples (2^?)"
  snap_eq_out : Subsystem  mask{nsamples=13}
      mask prompts: nsamples "Number of Samples (2^?)"
  snap_xaui0 : Subsystem  mask{nsamples=13}
      mask prompts: nsamples "Number of Samples (2^?)"
  sram_tvg : Subsystem
  sync_gen : Subsystem
  xaui_process : Subsystem
  wires:
  sync_gen/1(sync) -> [sync_gen]
  sync_gen/2(mrst) -> [mrst]
  [arm_rst] -> sync_gen/2(arm)
  [sync_rst] -> Logical7/2
  sync_gen/3(armed) -> [armed]
  Logical7/1 -> sync_gen/1(rst)
  [sync_adc0] -> Logical7/1
  [sync_adc1] -> Logical7/3
  quadc0/1 -> [adc0]
  quadc0/2 -> [adc1]
  quadc0/3 -> [adc2]
  quadc0/4 -> [adc3]
  quadc0/6 -> [sync_adc0]
  quadc1/1 -> [adc4]
  quadc1/2 -> [adc5]
  quadc1/3 -> [adc6]
  quadc1/4 -> [adc7]
  quadc1/6 -> [sync_adc1]
  Band-Limited White Noise/1 -> quadc1/4, quadc1/3, quadc1/2, quadc1/1, quadc0/4, quadc0/3, quadc0/2, quadc0/1
  Pulse Generator/1 -> quadc0/6, quadc1/6
  Constant1/1 -> quadc0/5, quadc1/5
  pfb_fir0/1(sync_out) -> [fft_sync]
  [adc0] -> ri_to_c/1
  [adc1] -> ri_to_c/2
  [sync_gen] -> pfb_fir0/1(sync)
  ri_to_c/1 -> pfb_fir0/2(pol1_in1)
  pfb_fir0/2(pol1_out1) -> c_to_ri/1
  c_to_ri/1 -> [pfb0]
  c_to_ri/2 -> [pfb1]
  [sync_gen] -> pfb_fir1/1(sync)
  ri_to_c1/1 -> pfb_fir1/2(pol1_in1)
  pfb_fir1/2(pol1_out1) -> c_to_ri1/1
  [sync_gen] -> pfb_fir2/1(sync)
  ri_to_c2/1 -> pfb_fir2/2(pol1_in1)
  pfb_fir2/2(pol1_out1) -> c_to_ri2/1
  [sync_gen] -> pfb_fir3/1(sync)
  ri_to_c3/1 -> pfb_fir3/2(pol1_in1)
  pfb_fir3/2(pol1_out1) -> c_to_ri3/1
  [adc2] -> ri_to_c1/1
  [adc3] -> ri_to_c1/2
  [adc4] -> ri_to_c2/1
  [adc5] -> ri_to_c2/2
  [adc6] -> ri_to_c3/1
  [adc7] -> ri_to_c3/2
  c_to_ri1/1 -> [pfb2]
  c_to_ri1/2 -> [pfb3]
  c_to_ri2/1 -> [pfb4]
  c_to_ri2/2 -> [pfb5]
  c_to_ri3/1 -> [pfb6]
  c_to_ri3/2 -> [pfb7]
  [adc0] -> calc_adc_sum_sq0/1(pol_in)
  calc_adc_sum_sq1/1(sum_sq) -> Reinterpret1/1
  calc_adc_sum_sq2/1(sum_sq) -> Reinterpret2/1
  calc_adc_sum_sq3/1(sum_sq) -> Reinterpret3/1
  edge_detect/1 -> calc_adc_sum_sq0/2(accum_rst), calc_adc_sum_sq1/2(accum_rst), calc_adc_sum_sq2/2(accum_rst), calc_adc_sum_sq3/2(accum_rst), calc_adc_sum_sq4/2(accum_rst), calc_adc_sum_sq5/2(accum_rst), calc_adc_sum_sq6/2(accum_rst), calc_adc_sum_sq7/2(accum_rst)
  [adc1] -> calc_adc_sum_sq1/1(pol_in)
  [adc2] -> calc_adc_sum_sq2/1(pol_in)
  [adc3] -> calc_adc_sum_sq3/1(pol_in)
  Counter/1 -> Slice16/1
  Slice16/1 -> edge_detect/1
  calc_adc_sum_sq4/1(sum_sq) -> Reinterpret4/1
  [adc4] -> calc_adc_sum_sq4/1(pol_in)
  calc_adc_sum_sq5/1(sum_sq) -> Reinterpret5/1
  calc_adc_sum_sq6/1(sum_sq) -> Reinterpret6/1
  calc_adc_sum_sq7/1(sum_sq) -> Reinterpret7/1
  [adc5] -> calc_adc_sum_sq5/1(pol_in)
  [adc6] -> calc_adc_sum_sq6/1(pol_in)
  [adc7] -> calc_adc_sum_sq7/1(pol_in)
  Reinterpret/1 -> [adc0_levels]
  Reinterpret1/1 -> [adc1_levels]
  Reinterpret2/1 -> [adc2_levels]
  Reinterpret3/1 -> [adc3_levels]
  Reinterpret4/1 -> [adc4_levels]
  Reinterpret5/1 -> [adc5_levels]
  Reinterpret6/1 -> [adc6_levels]
  Reinterpret7/1 -> [adc7_levels]
  Slice9/1 -> [use_sram_tvg]
  Slice7/1 -> [arm_rst]
  Slice6/1 -> [sync_rst]
  Slice21/1 -> [fft_shift]
  Delay1/1 -> Slice8/1, Slice7/1, Slice6/1, Slice21/1, Slice9/1
  Feng_ctl/1(data_out) -> Delay1/1
  [ctl_data] -> Feng_ctl/1(data_in)
  [ctl_addr] -> Feng_ctl/2(addr_in)
  [ctl_en] -> Feng_ctl/3(valid_in)
  xaui_process/2(data_out) -> [ctl_data]
  xaui_process/1(addr) -> [ctl_addr]
  Constant4/1 -> XAUI0/1
  Constant5/1 -> XAUI0/2
  XAUI0/5 -> neg_edge_ext0/1(in), Subsystem9/4(link_down)
  XAUI0/4 -> xaui_process/2(valid)
  neg_edge_ext0/1(out) -> [xaui_link_down], xaui_process/3(lnk_dn)
  xaui_process/3(we) -> [ctl_en]
  XAUI0/6 -> neg_edge_ext1/1(in), Subsystem9/5(tx_full)
  [sync_reorder] -> packetiser1/2(sync_in)
  [mrst] -> packetiser1/3(mrst_in)
  packetiser1/1(data_out) -> mux_adc_levels/1(data_in)
  packetiser1/2(valid_out) -> mux_adc_levels/2(valid_in)
  packetiser1/3(header_out) -> mux_adc_levels/3(header)
  packetiser1/4(eof) -> mux_adc_levels/4(eof)
  packetiser1/5(sync_out) -> mux_adc_levels/5(sync)
  mux_adc_levels/1(data_out) -> XAUI0/3, Subsystem9/1(data_in)
  mux_adc_levels/2(oob) -> XAUI0/4, Subsystem9/2(oob_in)
  mux_adc_levels/3(valid_out) -> XAUI0/5, Subsystem9/3(we_in)
  [mrst] -> mux_adc_levels/6(mrst)
  [adc0_levels] -> mux_adc_levels/7(adc_power0)
  [ant12_pol12_reorder] -> packetiser1/1(data_in)
  XAUI0/1 -> xaui_process/1(data_in)
  XAUI0/2 -> Terminator33/1
  XAUI0/3 -> Terminator34/1
  XAUI0/7 -> Terminator37/1
  [adc1_levels] -> mux_adc_levels/8(adc_power1)
  [adc2_levels] -> mux_adc_levels/9(adc_power2)
  [adc3_levels] -> mux_adc_levels/10(adc_power3)
  [adc4_levels] -> mux_adc_levels/11(adc_power4)
  [adc5_levels] -> mux_adc_levels/12(adc_power5)
  [adc6_levels] -> mux_adc_levels/13(adc_power6)
  [adc7_levels] -> mux_adc_levels/14(adc_power7)
  eq0/1(dout) -> [eq0]
  eq0/2(sync_out) -> [sync_rnd]
  [fft0] -> eq0/1(in)
  [eq_data_0] -> eq0/3(coeff)
  [eq_en_0] -> eq0/4(coeff_we)
  eq0/3(clip) -> [eq_clip0]
  eq_coeff1/1(data_out) -> [eq_data_1]
  eq_coeff1/2(addr_out) -> [eq_addr_1]
  eq_coeff1/3(valid_out) -> [eq_en_1]
  eq_coeff2/1(data_out) -> [eq_data_2]
  eq_coeff2/2(addr_out) -> [eq_addr_2]
  eq_coeff2/3(valid_out) -> [eq_en_2]
  [ctl_data] -> Slice18/1
  [ctl_addr] -> eq_coeff1/2(addr_in)
  [ctl_en] -> eq_coeff1/3(valid_in)
  [ctl_data] -> Slice19/1
  [ctl_addr] -> eq_coeff2/2(addr_in)
  [ctl_en] -> eq_coeff2/3(valid_in)
  Logical5/1 -> [eq_clip]
  Concat3/1 -> [eq_out]
  [eq_clip0] -> Logical5/1
  [eq_clip1] -> Logical5/2
  Slice18/1 -> eq_coeff1/1(data_in)
  Slice19/1 -> eq_coeff2/1(data_in)
  [sync_fft0] -> eq0/2(sync)
  [eq_addr_0] -> eq0/5(coeff_addr)
  [fft1] -> eq1/1(in)
  [sync_fft0] -> eq1/2(sync)
  [eq_data_1] -> eq1/3(coeff)
  [eq_en_1] -> eq1/4(coeff_we)
  [eq_addr_1] -> eq1/5(coeff_addr)
  [fft2] -> eq2/1(in)
  [sync_fft0] -> eq2/2(sync)
  [eq_data_2] -> eq2/3(coeff)
  [eq_en_2] -> eq2/4(coeff_we)
  [eq_addr_2] -> eq2/5(coeff_addr)
  [fft3] -> eq3/1(in)
  [sync_fft0] -> eq3/2(sync)
  [eq_data_3] -> eq3/3(coeff)
  [eq_en_3] -> eq3/4(coeff_we)
  [eq_addr_3] -> eq3/5(coeff_addr)
  eq1/1(dout) -> [eq1]
  eq1/2(sync_out) -> [eq_sync1]
  eq1/3(clip) -> [eq_clip1]
  eq2/1(dout) -> [eq2]
  eq2/2(sync_out) -> [eq_sync2]
  eq2/3(clip) -> [eq_clip2]
  eq3/1(dout) -> [eq3]
  eq3/2(sync_out) -> [eq_sync3]
  eq3/3(clip) -> [eq_clip3]
  [eq_clip2] -> Logical5/3
  [eq_clip3] -> Logical5/4
  [eq0] -> Concat3/1
  [eq1] -> Concat3/2
  [eq2] -> Concat3/3
  [eq3] -> Concat3/4
  eq_coeff3/1(data_out) -> [eq_data_3]
  eq_coeff3/2(addr_out) -> [eq_addr_3]
  eq_coeff3/3(valid_out) -> [eq_en_3]
  [ctl_data] -> Slice20/1
  [ctl_addr] -> eq_coeff3/2(addr_in)
  [ctl_en] -> eq_coeff3/3(valid_in)
  Slice20/1 -> eq_coeff3/1(data_in)
  eq_coeff0/1(data_out) -> [eq_data_0]
  eq_coeff0/2(addr_out) -> [eq_addr_0]
  eq_coeff0/3(valid_out) -> [eq_en_0]
  [ctl_data] -> Slice22/1
  [ctl_addr] -> eq_coeff0/2(addr_in)
  [ctl_en] -> eq_coeff0/3(valid_in)
  Slice22/1 -> eq_coeff0/1(data_in)
  [fft_sync] -> fft1/5
  [fft_shift] -> fft1/6
  fft1/1 -> [fft2]
  fft1/2 -> [fft3]
  fft1/3 -> [fft1_over]
  fft0/1 -> [fft0]
  fft0/2 -> [fft1]
  fft0/3 -> [fft0_over]
  fft0/4 -> [sync_fft0]
  pulse_ext2/1(out) -> led2_sync/1
  [sync_gen] -> pulse_ext2/1(in)
  [armed] -> led1_arm/1
  [xaui_link_down] -> led6_link_dn/1
  pulse_ext4/1(out) -> led4_eq_clip/1
  [eq_clip] -> pulse_ext4/1(in)
  [xaui_buffer_overflow] -> led7_xaui_overlfow/1
  calc_adc_sum_sq0/1(sum_sq) -> Reinterpret/1
  fft1/4 -> Terminator10/1
  quadc0/5 -> Terminator11/1
  quadc1/5 -> Terminator12/1
  led1_arm/1 -> Terminator27/1
  led4_eq_clip/1 -> Terminator2/1
  led2_sync/1 -> Terminator3/1
  led6_link_dn/1 -> Terminator4/1
  led7_xaui_overlfow/1 -> Terminator5/1
  Feng_ctl/2(valid_out) -> Terminator6/1
  [adc0] -> adc_clip_detect0/1(adc_in)
  [adc1] -> adc_clip_detect1/1(adc_in)
  [adc2] -> adc_clip_detect2/1(adc_in)
  [adc3] -> adc_clip_detect3/1(adc_in)
  [adc4] -> adc_clip_detect4/1(adc_in)
  [adc5] -> adc_clip_detect5/1(adc_in)
  [adc6] -> adc_clip_detect6/1(adc_in)
  [adc7] -> adc_clip_detect7/1(adc_in)
  adc_clip_detect0/1(clip) -> Logical1/1
  adc_clip_detect1/1(clip) -> Logical1/2
  adc_clip_detect2/1(clip) -> Logical1/3
  adc_clip_detect3/1(clip) -> Logical1/4
  adc_clip_detect4/1(clip) -> Logical1/5
  adc_clip_detect5/1(clip) -> Logical1/6
  adc_clip_detect6/1(clip) -> Logical1/7
  adc_clip_detect7/1(clip) -> Logical1/8
  Logical1/1 -> [adc_clip]
  [adc_clip] -> pulse_ext3/1(in)
  pulse_ext3/1(out) -> led5_adc_clip/1
  led5_adc_clip/1 -> Terminator1/1
  fft2x_tvg/1(dout) -> dbuf_ct_sram_fft_2x/1(din)
  fft2x_tvg/2(sync_out) -> dbuf_ct_sram_fft_2x/2(sync_in)
  sram_tvg/1(dout) -> one_ant_a_time/1(din)
  sram_tvg/2(sync_out) -> one_ant_a_time/2(sync)
  dbuf_ct_sram_fft_2x/1(out) -> sram_tvg/1(din)
  dbuf_ct_sram_fft_2x/2(sync_out) -> sram_tvg/2(sync)
  [use_sram_tvg] -> sram_tvg/3(use_tvg)
  one_ant_a_time/1(dout) -> [ant12_pol12_reorder]
  one_ant_a_time/2(sync_out) -> [sync_reorder]
  [use_fft_tvg] -> fft2x_tvg/3(use_tvg)
  [eq_out] -> fft2x_tvg/2(din)
  [sync_rnd] -> fft2x_tvg/1(sync)
  [pfb0] -> fft0/1
  [pfb2] -> fft0/2
  [pfb1] -> fft0/3
  [pfb3] -> fft0/4
  [fft_sync] -> fft0/5
  [fft_shift] -> fft0/6
  [pfb4] -> fft1/1
  [pfb6] -> fft1/2
  [pfb5] -> fft1/3
  [pfb7] -> fft1/4
  Slice8/1 -> [use_fft_tvg]
  neg_edge_ext1/1(out) -> [xaui_buffer_overflow]
  Subsystem9/1(data_out) -> snap_xaui0/1(data_in)
  Subsystem9/2(oob_out) -> snap_xaui0/2(oob_in)
  Subsystem9/3(we_out) -> snap_xaui0/3(we)
  Subsystem9/4(trig_out) -> snap_xaui0/4(trig)
  Subsystem9/5(stop) -> snap_xaui0/5(stop)
  [ant12_pol12_reorder] -> snap_ct_out/1(data_in)
  [sync_reorder] -> snap_ct_out/3(trig)
  Constant2/1 -> snap_ct_out/2(we)
  Constant3/1 -> snap_ct_out/4(stop)
  [eq_out] -> snap_eq_out/1(data_in)
  [sync_rnd] -> snap_eq_out/3(trig)
  Constant6/1 -> snap_eq_out/2(we)
  Constant7/1 -> snap_eq_out/4(stop)

== system i_128w_2k_10_r306f/Feng_ctl ==
  data_in : Inport  OutDataType=sfix(16)  OutScaling=2^0
  addr_in : Inport  Port=2  OutDataType=sfix(16)  OutScaling=2^0
  valid_in : Inport  Port=3  OutDataType=sfix(16)  OutScaling=2^0
  Constant : xbsIndex_r4/Constant  arith_type=Unsigned  const=addr_offset  n_bits=32  bin_pt=0  explicit_period=on  period=1  equ=P=C  opselect=C  inp2=PCIN>>17  opr=+  inp1=P  carry=CIN  dbl_ovrd=off  block_type=constant
  Logical : xbsIndex_r4/Logical  logical_function=AND  inputs=2  en=off  latency=0  precision=Full  arith_type=Unsigned  n_bits=8  bin_pt=2  align_bp=on  dbl_ovrd=off  block_type=logical
      settings: xl_area=[0, 0, 0, 0, 0, 0, 0]
  Register : xbsIndex_r4/Register  init=0  rst=off  en=on  dbl_ovrd=off  block_type=register
      settings: xl_area=[0, 0, 0, 0, 0, 0, 0]
  Register1 : xbsIndex_r4/Register  init=0  rst=off  en=off  dbl_ovrd=off  block_type=register
      settings: xl_area=[0, 0, 0, 0, 0, 0, 0]
  Register2 : xbsIndex_r4/Register  init=0  rst=off  en=off  dbl_ovrd=off  block_type=register
      settings: xl_area=[0, 0, 0, 0, 0, 0, 0]
  Register3 : xbsIndex_r4/Register  init=0  rst=off  en=off  dbl_ovrd=off  block_type=register
      settings: xl_area=[0, 0, 0, 0, 0, 0, 0]
  Relational : xbsIndex_r4/Relational  mode=a=b  en=off  latency=1  dbl_ovrd=off  block_type=relational
      settings: xl_area=[0, 0, 0, 0, 0, 0, 0]  block_version=10.1.3
  Slice22 : xbsIndex_r4/Slice  nbits=32  boolean_output=off  mode=Lower Bit Location + Width  bit1=0  base1=MSB of Input  bit0=0  base0=LSB of Input  dbl_ovrd=off  block_type=slice
      settings: infoedit="Extracts a given range of bits from each input sample and presents it at the output.  The output type is ordinarily unsigned with binary point at zero, but can be Boolean when the slice is one bit wide.<P><P>Hardware notes: In hardware this block costs nothing."  block_version=10.1.3
  data_out : Outport  OutDataType=sfix(16)  OutScaling=2^0
  valid_out : Outport  Port=2  OutDataType=sfix(16)  OutScaling=2^0
  wires:
  addr_in/1 -> Slice22/1
  Slice22/1 -> Relational/1
  Constant/1 -> Relational/2
  Relational/1 -> Logical/1
  valid_in/1 -> Register3/1
  Logical/1 -> Register/2, Register2/1
  Register/1 -> data_out/1
  data_in/1 -> Register1/1
  Register1/1 -> Register/1
  Register2/1 -> valid_out/1
  Register3/1 -> Logical/2

== system i_128w_2k_10_r306f/Subsystem9 ==
  data_in : Inport  OutDataType=sfix(16)  OutScaling=2^0
  oob_in : Inport  Port=2  OutDataType=sfix(16)  OutScaling=2^0
  we_in : Inport  Port=3  OutDataType=sfix(16)  OutScaling=2^0
  link_down : Inport  Port=4  OutDataType=sfix(16)  OutScaling=2^0
  tx_full : Inport  Port=5  OutDataType=sfix(16)  OutScaling=2^0
  Concat2 : xbsIndex_r4/Concat  num_inputs=3  dbl_ovrd=off  block_type=concat
      settings: block_version=10.1.3
  Constant9 : xbsIndex_r4/Constant  arith_type=Boolean  const=1  n_bits=1  bin_pt=0  explicit_period=on  period=1  equ=P=C  opselect=C  inp2=PCIN>>17  opr=+  inp1=P  carry=CIN  dbl_ovrd=off  block_type=constant
  Convert : xbsIndex_r4/Convert  arith_type=Unsigned  n_bits=32  bin_pt=0  quantization=Truncate  overflow=Wrap  latency=0  dbl_ovrd=off  pipeline=off  block_type=convert
      settings: block_version=10.1.3
  Delay{1..2,4,6} (4 alike) : xbsIndex_r4/Delay  en=off  latency=2  dbl_ovrd=off  reg_retiming=on  block_type=delay
      settings: xl_area=[0, 0, 0, 0, 0, 0, 0]
  Slice3 : xbsIndex_r4/Slice  nbits=1  boolean_output=on  mode=Lower Bit Location + Width  bit1=0  base1=MSB of Input  bit0=1  base0=LSB of Input  dbl_ovrd=off  block_type=slice
      settings: infoedit="Extracts a given range of bits from each input sample and presents it at the output.  The output type is ordinarily unsigned with binary point at zero, but can be Boolean when the slice is one bit wide.<P><P>Hardware notes: In hardware this block costs nothing."  block_version=10.1.3
  data_out : Outport  OutDataType=sfix(16)  OutScaling=2^0
  oob_out : Outport  Port=2  OutDataType=sfix(16)  OutScaling=2^0
  we_out : Outport  Port=3  OutDataType=sfix(16)  OutScaling=2^0
  trig_out : Outport  Port=4  OutDataType=sfix(16)  OutScaling=2^0
  stop : Outport  Port=5  OutDataType=sfix(16)  OutScaling=2^0
  wires:
  Delay1/1 -> data_out/1
  Delay4/1 -> Convert/1
  Delay6/1 -> trig_out/1
  oob_in/1 -> Slice3/1, Concat2/3
  Slice3/1 -> Delay6/1
  Delay2/1 -> we_out/1
  we_in/1 -> Delay2/1
  link_down/1 -> Concat2/2
  data_in/1 -> Delay1/1
  Concat2/1 -> Delay4/1
  Convert/1 -> oob_out/1
  Constant9/1 -> stop/1
  tx_full/1 -> Concat2/1
